simulink model "MEEN432_Project3_start"  (R2023b)
settings: Solver=VariableStepAuto  StartTime=0.0  StopTime=1369  RelTol=1e-3
values from neighbouring files (symbols this model uses):
  F_drag = 0    [Project3_init.m]
  I_w = 0    [Project3_init.m]
  m = 1000    [Project3_init.m]
  r = 0.3    [Project3_init.m]
  time = urban_time    [Project3_init.m]    (also in init_urban_epa.m = (0:1:1369)'; init_urban_epa_2cycle.m = (0:1:343)')
  urban_epa = [0 ... (first row only)    [init_urban_epa.m]    (also in init_urban_epa_2cycle.m)
libraries: slpidlib x1
settings Model: Creator=flare  LastModifiedBy=flare

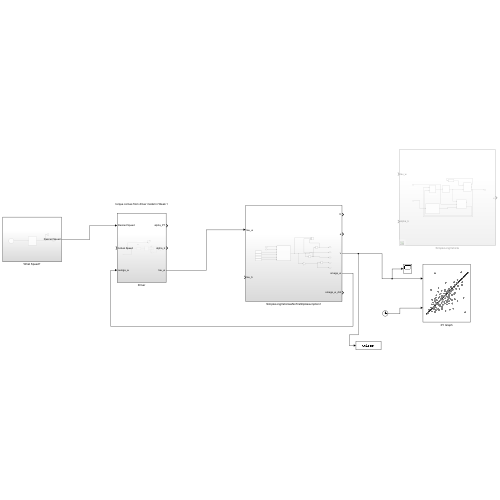
[thumbnail: Simulink's stored preview of the top-level diagram]
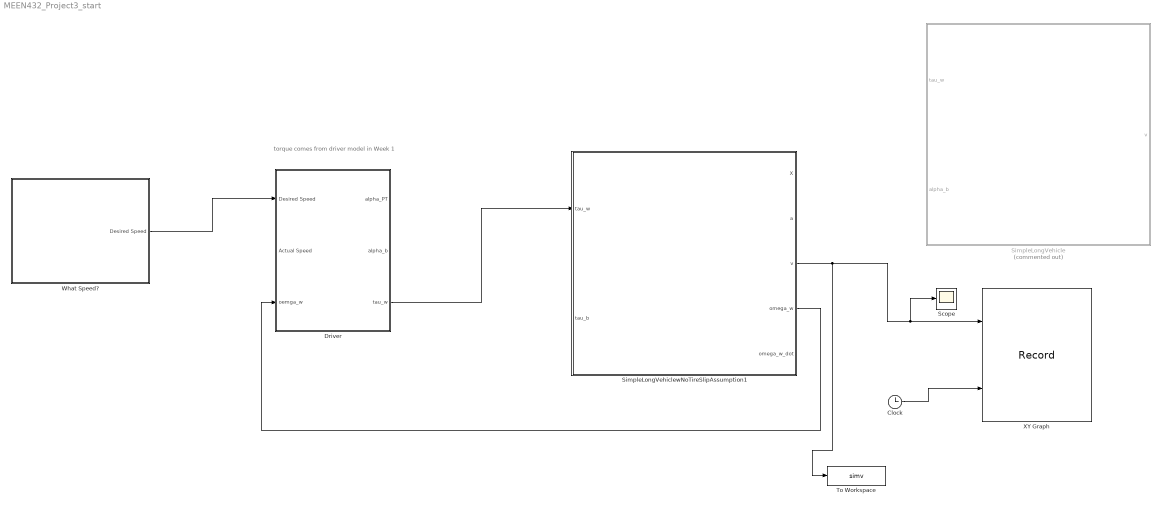
== system MEEN432_Project3_start ==
  note: torque comes from driver model in Week 1
  Clock : Clock
  Driver : Subsystem
  Scope : Scope
  SimpleLongVehicle : Subsystem  Commented=on
  SimpleLongVehiclewNoTireSlipAssumption1 : Subsystem
  To Workspace : ToWorkspace  VariableName=simv  SaveFormat=Timeseries  SampleTime=-1
  What Speed? : Subsystem
  XY Graph : Record  FileSettingsInternal="{\"entries\":[{\"content\":{\"excelSettings\":{\"content\":{},\"type\":\"Streamout.ExcelSettings\"}},\"type\":\"Streamout.FileSettingStorage\",\"uuid\":\"\"}],\"packageUris\":[\"http:\\/\\/schema.mathworks.com\\/mf0\\/streamout_blocks\\/R2020a\"],\"version\":\"1.0\"}"  Layout=[1 1]  SignalsInternal="{\"entries\":[{\"content\":{\"signals\":[{\"content\":{\"blockPath\":[],\"dimensions\":[1],\"domain\":\"\",\"lineColor\":\"#a2142f\",\"plots\":[1],\"port\":1,\"sid\":[\"\"],\"signalID\":526,\"signalName\":\"SimpleLongVehiclewNoTireSlipAssumption1:3\"},\"type\":\"RecordBlkView.Signal\",\"uuid\":\"\"},{\"content\":{\"blockPath\":[],\"dimensions\":[1],\"domain\":\"\",\"lineColor\":\"#139fff\",\"plots\":[1],\"port\":2,\"sid\":[\"\"],\"signalID\":530,\"signalName\":\"Clock\"},\"type\":\"RecordBlkView.Signal\",\"uuid\":\"\"}]},\"type\":\"RecordBlkView.InputSignals\",\"uuid\":\"\"}],\"packageUris\":[\"http:\\/\\/schema.mathworks.com\\/mf0\\/streamout_blocks\\/R2020a\"],\"version\":\"1.0\"}"  VisualizationBindings="{\"xyplotplugin\":{\"info\":[{\"series\":[{\"bindingParametersList\":[{\"parameter\":\"X-Axis\",\"signalID\":530,\"signalName\":\"Clock\"},{\"parameter\":\"Y-Axis\",\"signalID\":526,\"signalName\":\"SimpleLongVehiclewNoTireSlipAssumption1:3\"}],\"seriesID\":19400}],\"subplotID\":1}]}}"  CompatibilityTag=XY
  wires:
  What Speed?/1(Desired Speed) -> Driver/1(Desired Speed)
  Driver/3(tau_w) -> SimpleLongVehiclewNoTireSlipAssumption1/1(tau_w)
  SimpleLongVehiclewNoTireSlipAssumption1/3(v) -> To Workspace/1, Scope/1, XY Graph/1
  Clock/1 -> XY Graph/2
  SimpleLongVehiclewNoTireSlipAssumption1/4(omega_w) -> Driver/3(oemga_w)

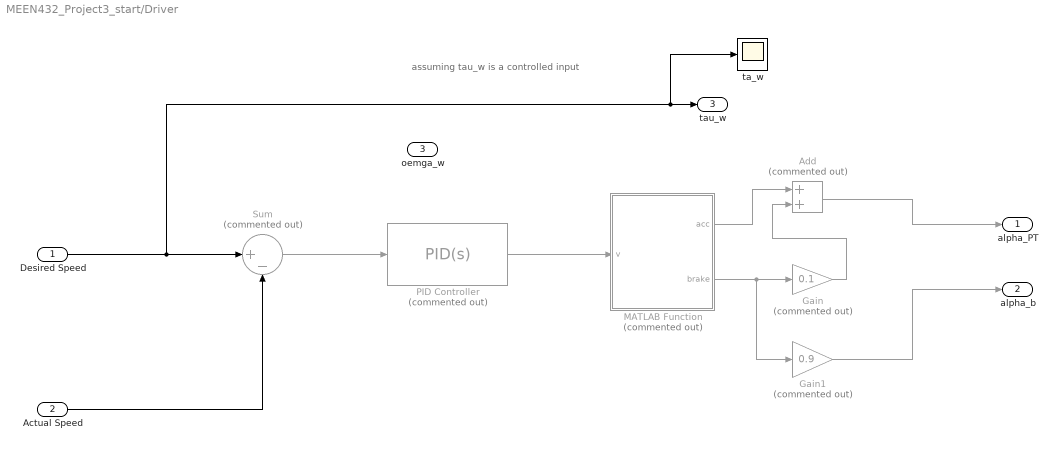
== system MEEN432_Project3_start/Driver ==
  note: assuming tau_w is a controlled input
  Desired Speed : Inport
  Actual Speed : Inport  Port=2
  oemga_w : Inport  Port=3
  Add : Sum  Commented=on
  Gain : Gain  Commented=on  Gain=0.1
  Gain1 : Gain  Commented=on  Gain=0.9
  MATLAB Function : MATLAB Function  Commented=on  TreatAsAtomicUnit=on
  PID Controller : slpidlib/PID Controller  Commented=on  Controller=PID  Form=Parallel  TimeDomain=Continuous-time  UseExternalTs=off  SampleTime=-1  IntegratorMethod=Forward Euler  FilterMethod=Forward Euler  ControllerParametersSource=internal  P=1  I=1  UseKiTs=off  D=0  N=100  UseFilter=on  TunerSelectOption=Transfer Function Based (PID Tuner App)  InitialConditionSource=internal  InitialConditionForIntegrator=0  InitialConditionForFilter=0  DifferentiatorICPrevScaledInput=0  ExternalReset=none  TrackingMode=off  Kt=1  LimitOutput=off  SatLimitsSource=internal  UpperSaturationLimit=inf  LowerSaturationLimit=-inf  LinearizeAsGain=on  AntiWindupMode=none  Kb=1  LimitIntegrator=off  UpperIntegratorSaturationLimit=inf  LowerIntegratorSaturationLimit=-inf  POutMin=[]  POutMax=[]  IOutMin=[]  IOutMax=[]  DOutMin=[]  DOutMax=[]  NOutMin=[]  NOutMax=[]  SumOutMin=[]  SumOutMax=[]  SaturationOutMin=[]  SaturationOutMax=[]  PParamMin=[]  PParamMax=[]  IParamMin=[]  IParamMax=[]  DParamMin=[]  DParamMax=[]  NParamMin=[]  NParamMax=[]  KbParamMin=[]  KbParamMax=[]  KtParamMin=[]  KtParamMax=[]  KbOutMin=[]  KbOutMax=[]  KtOutMin=[]  KtOutMax=[]  IntegratorOutMin=[]  IntegratorOutMax=[]  FilterOutMin=[]  FilterOutMax=[]  SumI1OutMin=[]  SumI1OutMax=[]  SumI2OutMin=[]  SumI2OutMax=[]  SumI3OutMin=[]  SumI3OutMax=[]  SumI4OutMin=[]  SumI4OutMax=[]  SumDOutMin=[]  SumDOutMax=[]  DifferentiatorOutMin=[]  DifferentiatorOutMax=[]  FilterDiffOutCoefMin=[]  FilterDiffOutCoefMax=[]  ReciprocalOutMin=[]  ReciprocalOutMax=[]  SumDenOutMin=[]  SumDenOutMax=[]  SumNumOutMin=[]  SumNumOutMax=[]  DivideOutMin=[]  DivideOutMax=[]  UdiffTsProdOutMin=[]  UdiffTsProdOutMax=[]  NTsProdOutMin=[]  NTsProdOutMax=[]  UintegralTsProdOutMin=[]  UintegralTsProdOutMax=[]  UngainTsProdOutMin=[]  UngainTsProdOutMax=[]  ClampingZeroOutDataTypeStr=Inherit: Inherit via back propagation  ClampingZeroOutMin=[]  ClampingZeroOutMax=[]  FilterDenConstantOutDataTypeStr=Inherit: Inherit via back propagation  FilterDenConstantOutMin=[]  FilterDenConstantOutMax=[]  PCopyOutDataTypeStr=Inherit: Inherit via back propagation  PCopyOutMin=[]  PCopyOutMax=[]  NCopyOutDataTypeStr=Inherit: Inherit via back propagation  NCopyOutMin=[]  NCopyOutMax=[]  IntegratorContinuousStateAttributes=''  IntegratorStateMustResolveToSignalObject=off  IntegratorRTWStateStorageClass=Auto  FilterContinuousStateAttributes=''  FilterStateMustResolveToSignalObject=off  FilterRTWStateStorageClass=Auto  ParallelPVariant=InternalParameters  IdealPVariant=Disabled  IVariant=InternalParameters  DVariant=InternalParameters  IntegratorVariant=Continuous  SatVariant=Disabled  AWVariant=Passthrough  PCopyVariant=Disabled  TRVariant=Disabled  FdbkBlocksVariant=Forward  IdealPFdbkVariant=Disabled  SatFdbkVariant=Disabled  DerivativeFilterVariant=ContFilter  NVariant=InternalParameters  NCopyVariant=Disabled  FilterICVariant=InternalICsFilter  IntegratorICVariant=InternalICs  ExternalResetVariant=Disabled  TRSumVariant=Passthrough  SumFdbkVariant=Disabled  SumVariant=Sum_PID  TsampFilterVariant=InternalTs  TsampNgainVariant=Passthrough  TsampIntegralVariant=Disabled_SignalSpec  ExternalSaturationOutDataTypeStr=Inherit: Same as second input
  Sum : Sum  Commented=on  Inputs=|+-
  ta_w : Scope
  alpha_PT : Outport
  alpha_b : Outport  Port=2
  tau_w : Outport  Port=3
  wires:
  Actual Speed/1 -> Sum/2
  Sum/1 -> PID Controller/1
  PID Controller/1 -> MATLAB Function/1(v)
  MATLAB Function/1(acc) -> Add/1
  MATLAB Function/2(brake) -> Gain1/1, Gain/1
  Gain/1 -> Add/2
  Gain1/1 -> alpha_b/1
  Add/1 -> alpha_PT/1
  Desired Speed/1 -> ta_w/1, tau_w/1, Sum/1

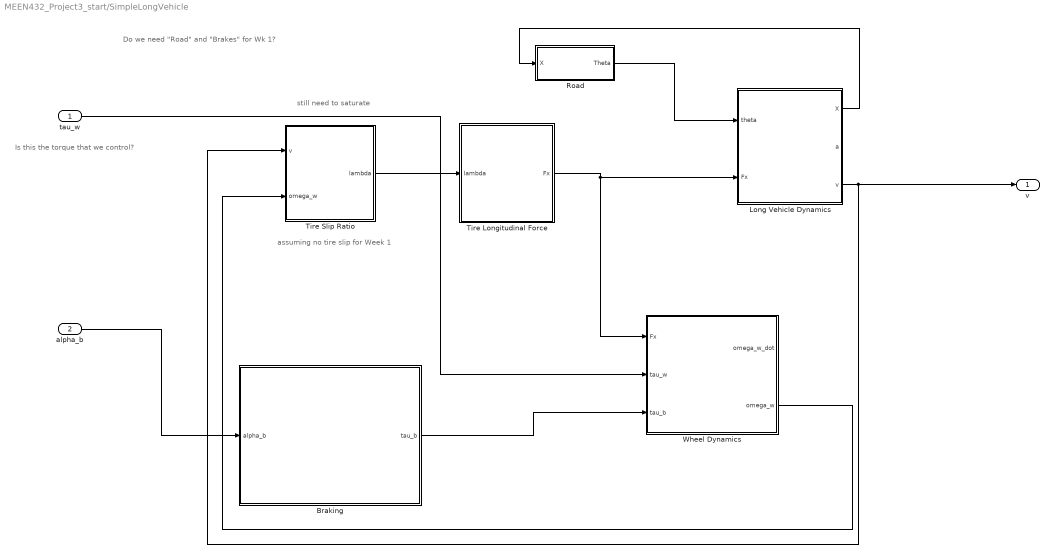
== system MEEN432_Project3_start/SimpleLongVehicle ==
  note: Is this the torque that we control?
  note: assuming no tire slip for Week 1
  note: still need to saturate
  note: Do we need "Road" and "Brakes" for Wk 1?
  tau_w : Inport
  alpha_b : Inport  Port=2
  Braking : Subsystem
  Long Vehicle Dynamics : Subsystem
  Road : Subsystem
  Tire Longitudinal Force : Subsystem
  Tire Slip Ratio : Subsystem
  Wheel Dynamics : Subsystem
  v : Outport
  wires:
  tau_w/1 -> Wheel Dynamics/2(tau_w)
  Tire Slip Ratio/1(lambda) -> Tire Longitudinal Force/1(lambda)
  alpha_b/1 -> Braking/1(alpha_b)
  Tire Longitudinal Force/1(Fx) -> Long Vehicle Dynamics/2(Fx), Wheel Dynamics/1(Fx)
  Road/1(Theta) -> Long Vehicle Dynamics/1(theta)
  Long Vehicle Dynamics/1(X) -> Road/1(X)
  Braking/1(tau_b) -> Wheel Dynamics/3(tau_b)
  Wheel Dynamics/2(omega_w) -> Tire Slip Ratio/2(omega_w)
  Long Vehicle Dynamics/3(v) -> Tire Slip Ratio/1(v), v/1

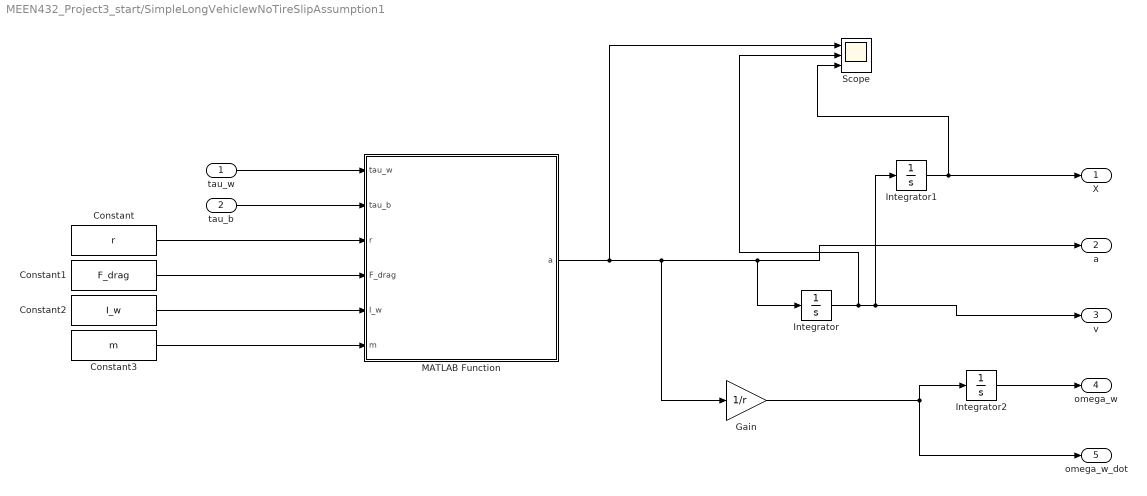
== system MEEN432_Project3_start/SimpleLongVehiclewNoTireSlipAssumption1 ==
  tau_w : Inport
  tau_b : Inport  Port=2
  Constant : Constant  Value=r
  Constant1 : Constant  Value=F_drag
  Constant2 : Constant  Value=I_w
  Constant3 : Constant  Value=m
  Gain : Gain  Gain=1/r
  Integrator : Integrator
  Integrator1 : Integrator
  Integrator2 : Integrator
  MATLAB Function : MATLAB Function  TreatAsAtomicUnit=on
  Scope : Scope  NumInputPorts=3
  X : Outport
  a : Outport  Port=2
  v : Outport  Port=3
  omega_w : Outport  Port=4
  omega_w_dot : Outport  Port=5
  wires:
  MATLAB Function/1(a) -> Scope/1, Gain/1, Integrator/1, a/1
  Integrator/1 -> Scope/2, Integrator1/1, v/1
  Integrator1/1 -> Scope/3, X/1
  Gain/1 -> Integrator2/1, omega_w_dot/1
  Integrator2/1 -> omega_w/1
  tau_w/1 -> MATLAB Function/1(tau_w)
  tau_b/1 -> MATLAB Function/2(tau_b)
  Constant/1 -> MATLAB Function/3(r)
  Constant1/1 -> MATLAB Function/4(F_drag)
  Constant2/1 -> MATLAB Function/5(I_w)
  Constant3/1 -> MATLAB Function/6(m)

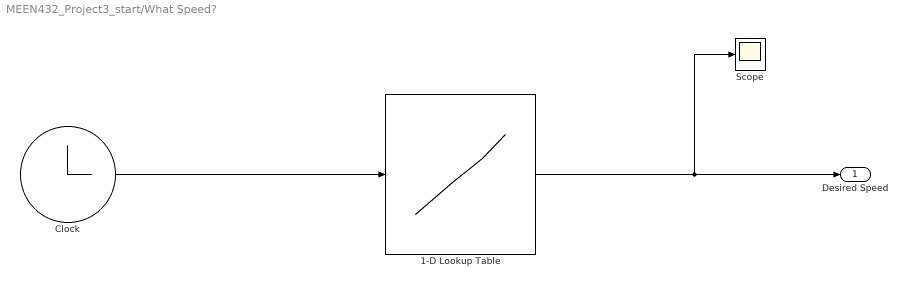
== system MEEN432_Project3_start/What Speed? ==
  1-D Lookup Table : Lookup_n-D  NumberOfTableDimensions=1  BreakpointsForDimension1=time  Table=urban_epa  InternalRulePriority=Speed  RndMeth=Simplest
  Clock : Clock
  Scope : Scope
  Desired Speed : Outport
  wires:
  Clock/1 -> 1-D Lookup Table/1
  1-D Lookup Table/1 -> Scope/1, Desired Speed/1

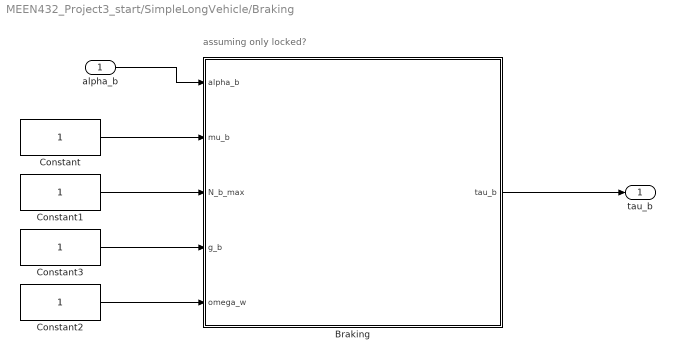
== system MEEN432_Project3_start/SimpleLongVehicle/Braking ==
  note: assuming only locked?
  alpha_b : Inport
  Braking : MATLAB Function  TreatAsAtomicUnit=on
  Constant{,1..3} (4 alike) : Constant
  tau_b : Outport
  wires:
  Braking/1(tau_b) -> tau_b/1
  alpha_b/1 -> Braking/1(alpha_b)
  Constant/1 -> Braking/2(mu_b)
  Constant1/1 -> Braking/3(N_b_max)
  Constant2/1 -> Braking/5(omega_w)
  Constant3/1 -> Braking/4(g_b)

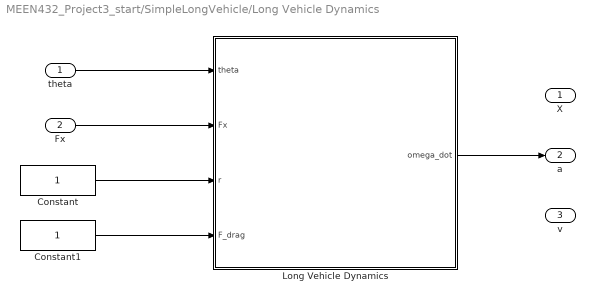
== system MEEN432_Project3_start/SimpleLongVehicle/Long Vehicle Dynamics ==
  theta : Inport
  Fx : Inport  Port=2
  Constant : Constant
  Constant1 : Constant
  Long Vehicle Dynamics : MATLAB Function  TreatAsAtomicUnit=on
  X : Outport
  a : Outport  Port=2
  v : Outport  Port=3
  wires:
  theta/1 -> Long Vehicle Dynamics/1(theta)
  Long Vehicle Dynamics/1(omega_dot) -> a/1
  Fx/1 -> Long Vehicle Dynamics/2(Fx)
  Constant/1 -> Long Vehicle Dynamics/3(r)
  Constant1/1 -> Long Vehicle Dynamics/4(F_drag)

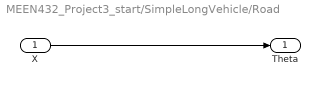
== system MEEN432_Project3_start/SimpleLongVehicle/Road ==
  X : Inport
  Theta : Outport
  wires:
  X/1 -> Theta/1

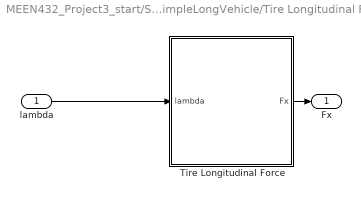
== system MEEN432_Project3_start/SimpleLongVehicle/Tire Longitudinal Force ==
  lambda : Inport
  Tire Longitudinal Force : MATLAB Function  TreatAsAtomicUnit=on
  Fx : Outport
  wires:
  lambda/1 -> Tire Longitudinal Force/1(lambda)
  Tire Longitudinal Force/1(Fx) -> Fx/1

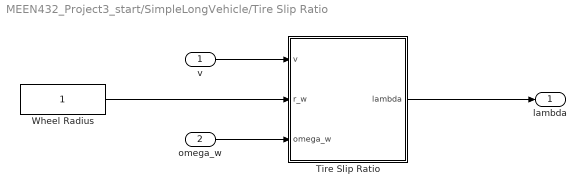
== system MEEN432_Project3_start/SimpleLongVehicle/Tire Slip Ratio ==
  v : Inport
  omega_w : Inport  Port=2
  Tire Slip Ratio : MATLAB Function  TreatAsAtomicUnit=on
  Wheel Radius : Constant
  lambda : Outport
  wires:
  v/1 -> Tire Slip Ratio/1(v)
  Tire Slip Ratio/1(lambda) -> lambda/1
  omega_w/1 -> Tire Slip Ratio/3(omega_w)
  Wheel Radius/1 -> Tire Slip Ratio/2(r_w)

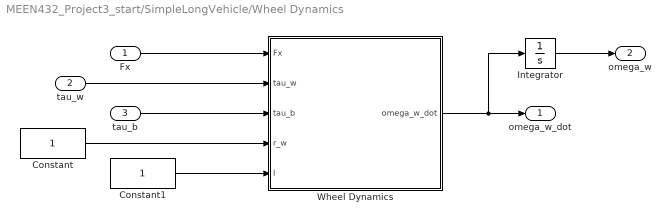
== system MEEN432_Project3_start/SimpleLongVehicle/Wheel Dynamics ==
  Fx : Inport
  tau_w : Inport  Port=2
  tau_b : Inport  Port=3
  Constant : Constant
  Constant1 : Constant
  Integrator : Integrator
  Wheel Dynamics : MATLAB Function  TreatAsAtomicUnit=on
  omega_w_dot : Outport
  omega_w : Outport  Port=2
  wires:
  Fx/1 -> Wheel Dynamics/1(Fx)
  tau_w/1 -> Wheel Dynamics/2(tau_w)
  tau_b/1 -> Wheel Dynamics/3(tau_b)
  Wheel Dynamics/1(omega_w_dot) -> Integrator/1, omega_w_dot/1
  Constant/1 -> Wheel Dynamics/4(r_w)
  Constant1/1 -> Wheel Dynamics/5(I)
  Integrator/1 -> omega_w/1

== matlab function MEEN432_Project3_start/SimpleLongVehicle/Tire Longitudinal Force/Tire Longitudinal Force ==
  data: lambda input; Fx output
function Fx = fcn(lambda)

y = u;

== matlab function MEEN432_Project3_start/SimpleLongVehicle/Tire Slip Ratio/Tire Slip Ratio ==
  data: v input; lambda output; r_w input; omega_w input
function lambda = fcn(v, r_w, omega_w)

if (r_w*omega_w - v) >= 0
    lambda = (r_w*omega_w - v)/(r_w*omega_w);
else
    lambda = (r_w*omega_w - v)/v;
end

== matlab function MEEN432_Project3_start/SimpleLongVehicle/Wheel Dynamics/Wheel Dynamics ==
  data: Fx input; omega_w_dot output; tau_w input; tau_b input; r_w input; I input
function omega_w_dot = fcn(Fx, tau_w, tau_b, r_w, I)

y = u;

== matlab function MEEN432_Project3_start/SimpleLongVehicle/Long Vehicle Dynamics/Long Vehicle Dynamics ==
  data: theta input; omega_dot output; Fx input; r input; F_drag input
function omega_dot = fcn(theta, Fx, r, F_drag)
g = 9.81;
omega_dot = (Fx*r - F_drag*r - m*g*r*sin(theta))/(m*r^2);

== matlab function MEEN432_Project3_start/SimpleLongVehicle/Braking/Braking ==
  data: alpha_b input; mu_b input; tau_b output; N_b_max input; g_b input; omega_w input
function tau_b = fcn(alpha_b, mu_b, N_b_max, g_b, omega_w)

N_b = alpha_b * N_b_max;

tau_b = mu_b * N_b * g_b * sign(omega_w);

== matlab function MEEN432_Project3_start/Driver/MATLAB Function ==
  data: v input; acc output; brake output
function [acc, brake] = fcn(v)

if v > 0
    acc = v;
    brake = 0;
elseif u < 0
    acc = 0;
    brake = v;
else
    acc = 0;
    brake = 0;
end

== matlab function MEEN432_Project3_start/SimpleLongVehiclewNoTireSlipAssumption1/MATLAB Function ==
  data: tau_w input; a output; tau_b input; r input; F_drag input; I_w input; m input
function a = fcn(tau_w, tau_b, r, F_drag, I_w, m)
theta = 90;
g = 9.81;

num = ((tau_w - tau_b) / r) - F_drag;
a = num / ((I_w / r^2) + m);
